simulink model "HelicopterRealUnitTest"  (R2023a)
settings: Solver=ode4  StartTime=0.0  StopTime=inf  FixedStep=0.1  RelTol=1e-3
undefined symbols (not defined in the file or in its folder): daq
libraries: simulink_extras x4, daqlib x2
settings Model: Creator=Jardar Fagerlund  LastModifiedBy=Jardar Fagerlund

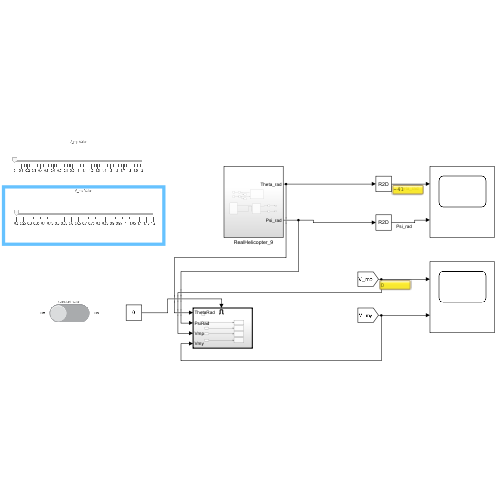
[thumbnail: Simulink's stored preview of the top-level diagram]
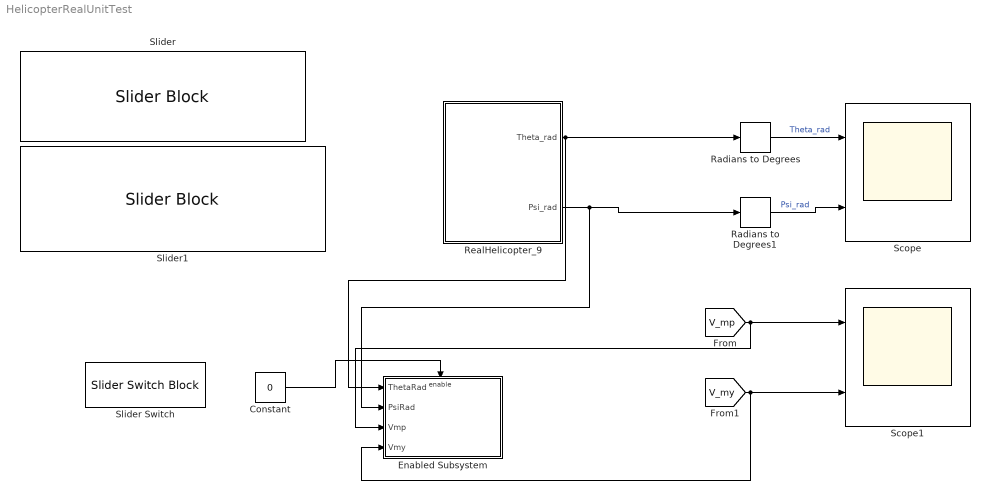
== system HelicopterRealUnitTest ==
  Constant : Constant  Value=0
  Enabled Subsystem : Subsystem  TreatAsAtomicUnit=on
  Radians to Degrees : simulink_extras/Transformations/Radians to Degrees
  Radians to Degrees1 : simulink_extras/Transformations/Radians to Degrees
  RealHelicopter_9 : Subsystem
  Scope : Scope  NumInputPorts=2
  Scope1 : Scope  NumInputPorts=2
  Slider : SliderBlock  ScaleMax=2
  Slider Switch : SliderSwitchBlock
      settings: Values={{'Off', 'On'}, [0 1]}
  Slider1 : SliderBlock  ScaleMin=0.2  ScaleMax=1.2
  wires:
  Radians to Degrees1/1 -> Scope/2  "Psi_rad"
  RealHelicopter_9/2(Psi_rad) -> Enabled Subsystem/2(PsiRad), Radians to Degrees1/1
  RealHelicopter_9/1(Theta_rad) -> Enabled Subsystem/1(ThetaRad), Radians to Degrees/1
  Radians to Degrees/1 -> Scope/1  "Theta_rad"
  [V_mp] -> Enabled Subsystem/3(Vmp), Scope1/1
  [V_my] -> Enabled Subsystem/4(Vmy), Scope1/2
  Constant/1 -> Enabled Subsystem/Enable

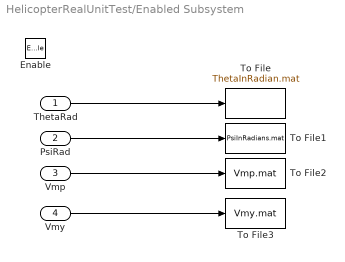
== system HelicopterRealUnitTest/Enabled Subsystem ==
  ThetaRad : Inport
  PsiRad : Inport  Port=2
  Vmp : Inport  Port=3
  Vmy : Inport  Port=4
  Enable : EnablePort
  To File : ToFile  Filename=ThetaInRadian.mat  MatrixName=Theta  SaveFormat=Timeseries  SampleTime=0.1
  To File1 : ToFile  Filename=PsiInRadians.mat  MatrixName=Psi  SaveFormat=Timeseries  SampleTime=0.1
  To File2 : ToFile  Filename=Vmp.mat  MatrixName=Vmp  SaveFormat=Timeseries  SampleTime=0.1
  To File3 : ToFile  Filename=Vmy.mat  MatrixName=Vmy  SaveFormat=Timeseries  SampleTime=0.1
  wires:
  ThetaRad/1 -> To File/1
  Vmy/1 -> To File3/1
  Vmp/1 -> To File2/1
  PsiRad/1 -> To File1/1

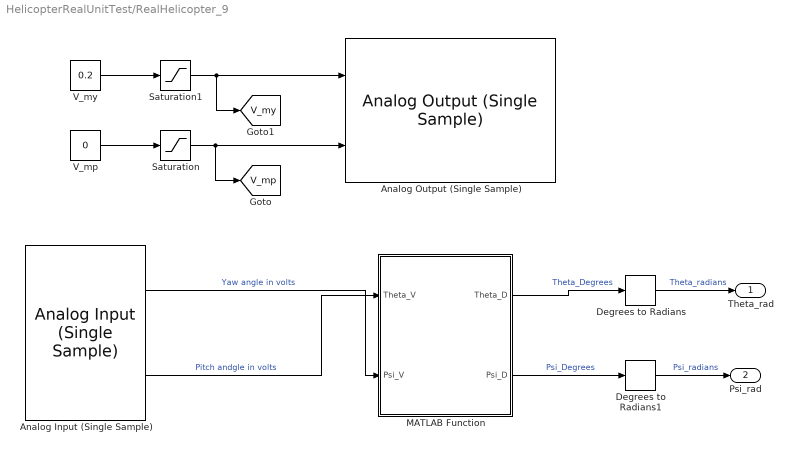
== system HelicopterRealUnitTest/RealHelicopter_9 ==
  Analog Input (Single Sample) : daqlib/Analog Input (Single Sample)  DeviceMenu=ni Dev1 (USB-6001)  Device=ni Dev1 (USB-6001)  ObjConstructor=daq.createSession('ni')  BlockSampleTime=0.1  NChannelsSelected=2  Channels=1$ai0$$Dev1$1$1$1$1$#1$ai1$$Dev1$1$1$1$1$#0$ai2$$Dev1$1$1$2$1$#0$ai3$$Dev1$1$1$2$1$#0$ai4$$Dev1$1$1$1$1$#0$ai5$$Dev1$1$1$1$1$#0$ai6$$Dev1$1$1$1$1$#0$ai7$$Dev1$1$1$1$1$#  NPorts=1 per channel  OutputTimestamp=off
  Analog Output (Single Sample) : daqlib/Analog Output (Single Sample)  DeviceMenu=ni Dev1 (USB-6001)  Device=ni Dev1 (USB-6001)  ObjConstructor=daq.createSession('ni')  NChannelsSelected=2  Channels=1$ao0$$Dev1$1$1$N/A$#1$ao1$$Dev1$1$1$N/A$#  NPorts=1 per channel  BlockSampleTime=0.1
  Degrees to Radians : simulink_extras/Transformations/Degrees to Radians
  Degrees to Radians1 : simulink_extras/Transformations/Degrees to Radians
  MATLAB Function : MATLAB Function  TreatAsAtomicUnit=on
  Saturation : Saturate  UpperLimit=3  LowerLimit=0
  Saturation1 : Saturate  UpperLimit=3  LowerLimit=0
  V_mp : Constant  Value=0
  V_my : Constant  Value=0.2
  Theta_rad : Outport
  Psi_rad : Outport  Port=2
  tag scope: V_mp=global, V_my=global
  wires:
  Saturation1/1 -> [V_my], Analog Output (Single Sample)/1
  Saturation/1 -> [V_mp], Analog Output (Single Sample)/2
  Analog Input (Single Sample)/1 -> MATLAB Function/2(Psi_V)  "Yaw angle in volts"
  Analog Input (Single Sample)/2 -> MATLAB Function/1(Theta_V)  "Pitch andgle in volts"
  MATLAB Function/1(Theta_D) -> Degrees to Radians/1  "Theta_Degrees"
  MATLAB Function/2(Psi_D) -> Degrees to Radians1/1  "Psi_Degrees"
  Degrees to Radians/1 -> Theta_rad/1  "Theta_radians"
  Degrees to Radians1/1 -> Psi_rad/1  "Psi_radians"
  V_my/1 -> Saturation1/1
  V_mp/1 -> Saturation/1

== matlab function HelicopterRealUnitTest/RealHelicopter_9/MATLAB Function ==
  data: Theta_V input; Theta_D output; Psi_V input; Psi_D output
function [Theta_D, Psi_D] = VoltageToDegrees(Theta_V, Psi_V)

Theta_D = 90*Theta_V/5 - 45;
Psi_D = 180*Psi_V/5;
